simulink model "lqr"  (R2022a)
settings: Solver=VariableStepAuto  StartTime=0.0  StopTime=20  RelTol=1e-3
values from neighbouring files (symbols this model uses):
  A = [0 1; -15.3 -0.2142]    [PID.m]    (also in Pasos_lqr.m = [0 1;-15.3 -0.3312])
  B = [0;5.218]    [PID.m]    (also in Pasos_lqr.m = [0; 5.218])
  C = [1 0]    [PID.m]    (also in Pasos_lqr.m)
  K = Ks(:,1:2)    [Pasos_lqr.m]
  Ki = PIDSYS.Ki    [PID.m]    (also in Pasos_lqr.m = -Ks(:,3))
settings Model: Creator=de-je  LastModifiedBy=carlo
settings SolverCC: AlgebraicLoopSolver=TrustRegion
settings DebuggingCC: UnconnectedInputMsg=warning  UnconnectedOutputMsg=warning  UnconnectedLineMsg=warning  SFMachineParentedDataDiag=warning

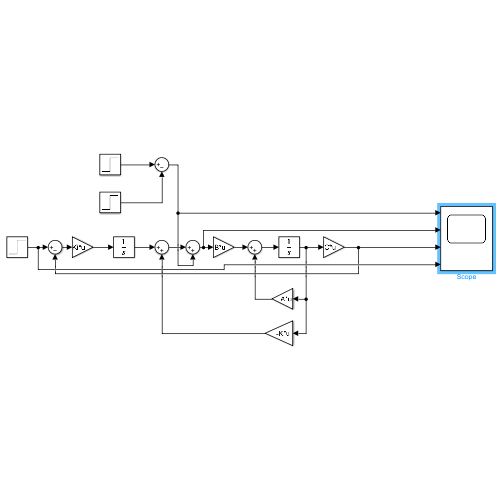
[thumbnail: Simulink's stored preview of the top-level diagram]
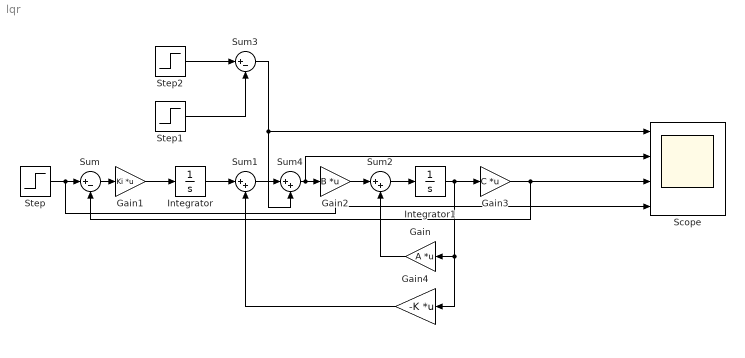
== system lqr ==
  Gain : Gain  Gain=A  Multiplication=Matrix(K*u)
  Gain1 : Gain  Gain=Ki  Multiplication=Matrix(K*u)
  Gain2 : Gain  Gain=B  Multiplication=Matrix(K*u)
  Gain3 : Gain  Gain=C  Multiplication=Matrix(K*u)
  Gain4 : Gain  Gain=-K  Multiplication=Matrix(K*u)
  Integrator : Integrator
  Integrator1 : Integrator
  Scope : Scope  NumInputPorts=4
  Step : Step  After=0.6  SampleTime=0
  Step1 : Step  Time=17  After=0.05  SampleTime=0
  Step2 : Step  Time=15  After=0.05  SampleTime=0
  Sum : Sum  Inputs=|+-
  Sum1 : Sum  Inputs=|++
  Sum2 : Sum  Inputs=|++
  Sum3 : Sum  Inputs=|+-
  Sum4 : Sum  Inputs=|++
  wires:
  Step/1 -> Scope/4, Sum/1
  Gain2/1 -> Sum2/1
  Sum2/1 -> Integrator1/1
  Integrator1/1 -> Gain4/1, Gain/1, Gain3/1
  Gain3/1 -> Sum/2, Scope/3
  Gain/1 -> Sum2/2
  Gain4/1 -> Sum1/2
  Sum/1 -> Gain1/1
  Integrator/1 -> Sum1/1
  Gain1/1 -> Integrator/1
  Step2/1 -> Sum3/1
  Step1/1 -> Sum3/2
  Sum1/1 -> Sum4/1
  Sum4/1 -> Scope/2, Gain2/1
  Sum3/1 -> Scope/1, Sum4/2
